simulink model "control_ident_31"  (Simulink 4.00)
settings: Solver=ode45  StartTime=0.0  StopTime=10.0  RelTol=1e-3
values from neighbouring files (symbols this model uses):
  A = conv([1,-(0.8+j*0.5)],[1,-(0.8-j*0.5)])    [anfangsbed1.m]    (also in control_ident2.m; control_ident3.m; control_ident31.m; ident_verg1.m = conv([1, -0.6+j*0.3],[1, -0.6-j*0.3]))
  a = 1    [control_ident3.m]    (also in control_ident31.m; ident_1.m = my_sys1.den{1,:}; ident_2.m = my_sys1.den{1,:}; ident_3.m = my_sys1.den{1,:})
  C = [1,1]    [anfangsbed1.m]    (also in control_ident2.m; control_ident3.m; control_ident31.m; ident_verg1.m = [1, -1, 0.2])
  Ts = 0.5    [anfangsbed1.m]    (also in control_ident2.m; control_ident3.m; control_ident31.m; delay_1.m)
settings Model: LastModifiedBy=Administrator  BlockReductionOpt=off

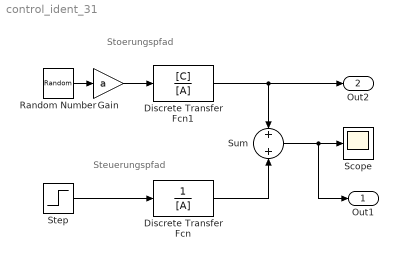
== system control_ident_31 ==
  note: Steuerungspfad
  note: Stoerungspfad
  Discrete Transfer Fcn : DiscreteTransferFcn  Numerator=[1]  Denominator=[A]  SampleTime=Ts  Realization=auto
  Discrete Transfer Fcn1 : DiscreteTransferFcn  Numerator=[C]  Denominator=[A]  SampleTime=Ts  Realization=auto
  Gain : Gain  Gain=a  Multiplication=Element-wise(K.*u)  SaturateOnIntegerOverflow=on
  Random Number : RandomNumber  Mean=0  Variance=1  Seed=0  SampleTime=0
  Scope : Scope
      settings: TimeRange=auto  YMin=-5  YMax=5  SaveToWorkspace=off  SaveName=ScopeData  LimitDataPoints=on  MaxDataPoints=5000
  Step : Step  Time=0  Before=0  After=1  SampleTime=0
  Sum : Sum  Inputs=+|+  SaturateOnIntegerOverflow=on
  Out1 : Outport  Port=1
  Out2 : Outport  Port=2
  wires:
  Step/1 -> Discrete Transfer Fcn/1
  Random Number/1 -> Gain/1
  Sum/1 -> Scope/1, Out1/1
  Gain/1 -> Discrete Transfer Fcn1/1
  Discrete Transfer Fcn/1 -> Sum/2
  Discrete Transfer Fcn1/1 -> Sum/1, Out2/1
